simulink model "Pendulum"  (R2013a)
settings: Solver=ode1  SolverMode=SingleTasking  StartTime=0.0  StopTime=inf  FixedStep=0.01  RelTol=1e-3
InitFcn:
  | fuzzycontroller1=readfis('fuzzy1.fis');
  | fuzzycontroller2=readfis('fuzzy2.fis');
  | fuzzypid=readfis('fuzzy3.fis');
libraries: neural x91, fuzblock x9
(part 1 of 2)
settings Model: Creator=Administrator  LastModifiedBy=Administrator

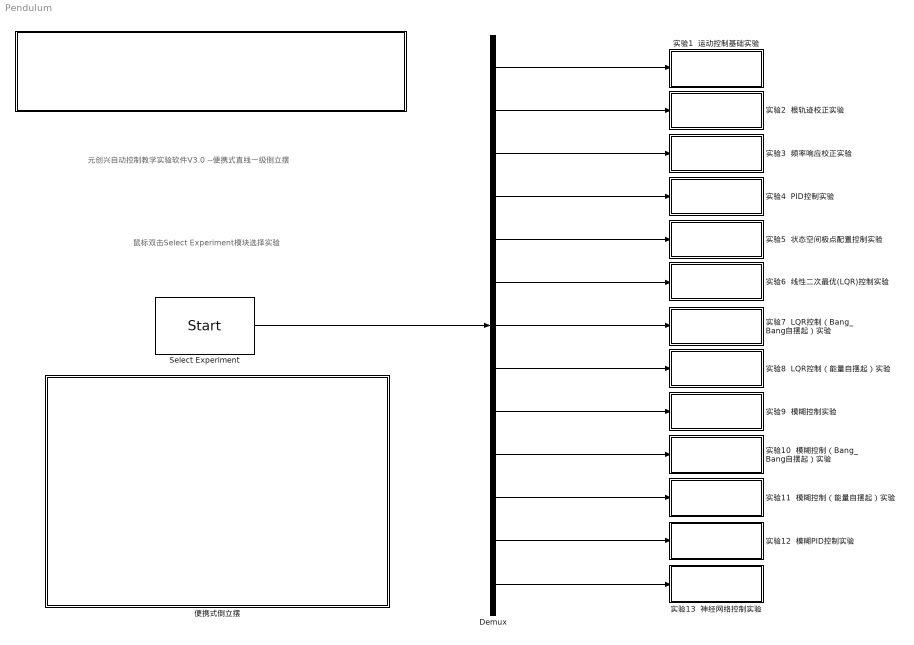
== system Pendulum ==
  note: 鼠标双击Select Experiment模块选择实验
  note: 元创兴自动控制教学实验软件V3.0
      | --便携式直线一级倒立摆
  " " : Subsystem  mask(便携式倒立摆系统实时控制程序){}
      mask help:
      | 程序版本：REI-PD-M-V3.0
      | 开发环境：Matlab2013a Simulink
      | 操作系统：Windows 7 旗舰版 32位
      | 深圳市元创兴科技有限公司
      | Copyright (C) 2015
      | 技术支持：0755-86000801
      mask Display: image('logo.PNG')
  Demux : Demux  Outputs=13
  Select Experiment : S-Function  FunctionName=Start  Parameters=ExpNum  EnableBusSupport=off  mask(SelectExperiment){ExpNum=7}
      mask prompts: ExpNum "选择实验编号："
      mask help:
      | 元创兴便携式倒立摆simulink模块：
      |
      | 便携式倒立摆可以开展以下实验：
      | 1.运动控制基础实验（编码器原理及电机运动测试）；
      | 2.根轨迹校正实验；
      | 3.频率响应校正实验；
      | 4.PID控制实验；
      | 5.状态空间极点配置控制实验；
      | 6.线性二次型最优控制实验（LQR）；
      | 7.LQR控制（Bang_Bang自摆起）实验；
      | 8.LQR控制（能量自摆起）实验；
      | 9.模糊控制实验；
      | 10.模糊控制（Bang_Bang自摆起）实验；
      | 11.模糊控制（能量自摆起）实验；
      | 12.模糊PID控制实验；
      | 13.神经网络控制实验；
      |
      | 选择实验编号后再点选启动开始实验，如果需要开展其他实验，请先停止实验后再选择。
      mask TypeOptions ExpNum: 1 | 2 | 3 | 4 | 5 | 6 | 7 | 8 | 9 | 10 | 11 | 12 | 13
      mask Display: fprintf('实验%d',ExpNum)
  便携式倒立摆 : Subsystem
      mask Display: image('Reinovo.jpg')
  实验1  运动控制基础实验 : Subsystem
  实验10  模糊控制（Bang_Bang自摆起）实验 : Subsystem  TreatAsAtomicUnit=on
  实验11  模糊控制（能量自摆起）实验 : Subsystem  TreatAsAtomicUnit=on
  实验12  模糊PID控制实验 : Subsystem  TreatAsAtomicUnit=on
  实验13  神经网络控制实验 : Subsystem  TreatAsAtomicUnit=on
  实验2  根轨迹校正实验 : Subsystem
  实验3  频率响应校正实验 : Subsystem
  实验4  PID控制实验 : Subsystem
  实验5  状态空间极点配置控制实验 : Subsystem
  实验6  线性二次最优(LQR)控制实验 : Subsystem
  实验7  LQR控制（Bang_Bang自摆起）实验 : Subsystem
  实验8  LQR控制（能量自摆起）实验 : Subsystem
  实验9  模糊控制实验 : Subsystem  TreatAsAtomicUnit=on
  wires:
  Demux/1 -> 实验1  运动控制基础实验/Enable
  Demux/2 -> 实验2  根轨迹校正实验/Enable
  Demux/3 -> 实验3  频率响应校正实验/Enable
  Demux/4 -> 实验4  PID控制实验/Enable
  Demux/5 -> 实验5  状态空间极点配置控制实验/Enable
  Demux/6 -> 实验6  线性二次最优(LQR)控制实验/Enable
  Demux/7 -> 实验7  LQR控制（Bang_Bang自摆起）实验/Enable
  Demux/8 -> 实验8  LQR控制（能量自摆起）实验/Enable
  Select Experiment/1 -> Demux/1
  Demux/9 -> 实验9  模糊控制实验/Enable
  Demux/10 -> 实验10  模糊控制（Bang_Bang自摆起）实验/Enable
  Demux/11 -> 实验11  模糊控制（能量自摆起）实验/Enable
  Demux/12 -> 实验12  模糊PID控制实验/Enable
  Demux/13 -> 实验13  神经网络控制实验/Enable

== system Pendulum/  ==

== system Pendulum/便携式倒立摆 ==

== system Pendulum/实验1  运动控制基础实验 ==
  note: 数值输入范围[-0.2~0.2] 单位m
  note: 即电机转动一圈反馈回来的脉冲数为4000
  note: 实际脉冲数
  note: 目标脉冲数
  note: 实际位移量
  note: 目标位移量
  note: 小车位置脉冲
  note: 摆杆位置脉冲
  note: 实验1 运动控制基础实验
  note: 运行前请留意小车目标位移量设置
  note: 注意：实验开始前先将小车移至导轨中间位置
  note: 1.光电编码器认知实验部分
  note: 1.摆杆编码器为500线，四倍频：500*4=2000，即摆杆旋转一圈反馈回来的脉冲数为2000
  note: 2.直流伺服电机位置控制实验
  note: 2. 电机编码器为1000线，四倍频：1000*4=4000，
  note: 转换关系：电机直径=0.0355m,周长= 0.0355*3.141592=0.1117465m,
      |   即电机转动一周小车移动的位移量=0.1117465m
  note: 电机脉冲当量=0.1117465m/4000pulse
  Enable : EnablePort
  " " : Display
  Demux : Demux  Outputs=2
  Mux : Mux  Inputs=2
  Mux1 : Mux
  小车目标位移量 : Constant  Value=0.13
  小车移动至目标位置 : S-Function  FunctionName=MoveCartPos  EnableBusSupport=off
  数字显示 : Display
  显示摆杆脉冲和角度 : Scope  NumInputPorts=2
      settings: RequirementInfo="{}  %GIDa_b12c0a95_567d_4469_aa8f_37c49eb9258f"  YMin=-5~-5  YMax=5~5
  读取两路脉冲信号 : S-Function  FunctionName=Readtwochannelpulse  Parameters=1  EnableBusSupport=off
  转换为位移 : Gain  Gain=0.1117465/4000
  转换为弧度 : Gain  Gain=2*3.1415926/2000
  转换为脉冲数 : Gain  Gain=4000/0.1117465
  wires:
  Demux/2 -> Mux/1, 显示摆杆脉冲和角度/1, 转换为弧度/1
  Demux/1 -> Mux1/4, 转换为位移/1
  读取两路脉冲信号/1 -> Demux/1
  转换为弧度/1 -> Mux/2, 显示摆杆脉冲和角度/2
  Mux/1 -> 数字显示/1
  Mux1/1 -> " "/1
  转换为位移/1 -> Mux1/2
  转换为脉冲数/1 -> Mux1/3
  小车目标位移量/1 -> 转换为脉冲数/1, Mux1/1, 小车移动至目标位置/1

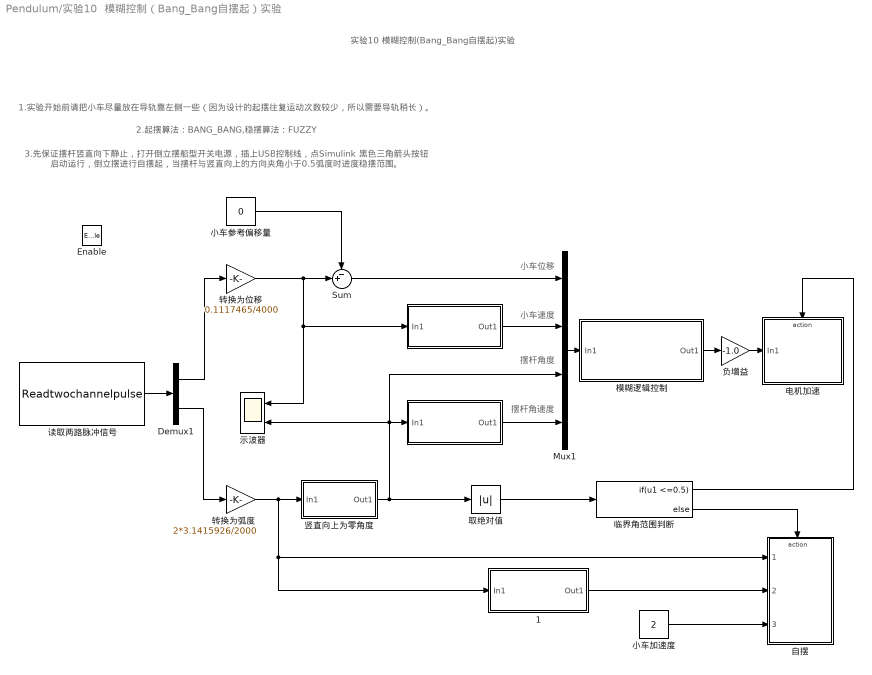
== system Pendulum/实验10  模糊控制（Bang_Bang自摆起）实验 ==
  note: 摆杆角速度
  note: 摆杆角度
  note: 小车速度
  note: 小车位移
  note: 实验10 模糊控制(Bang_Bang自摆起)实验
  note: 1.实验开始前请把小车尽量放在导轨靠左侧一些（因为设计的起摆往复运动次数较少，所以需要导轨稍长）。
  note: 3.先保证摆杆竖直向下静止，打开倒立摆船型开关电源，插上USB控制线，点Simulink 黑色三角箭头按钮
      | 启动运行，倒立摆进行自摆起，当摆杆与竖直向上的方向夹角小于0.5弧度时进度稳摆范围。
  note: 2.起摆算法：BANG_BANG,稳摆算法：FUZZY
  Enable : EnablePort
  " " : Subsystem
      mask help: 对摆杆角度求导得到摆杆角速度
      mask Display: disp('计算摆杆角速度')
  "  " : Subsystem
      mask help: 对小车位移求导得到小车速度
      mask Display: disp('计算小车速度')
  " 1" : Subsystem
      mask help: 对摆杆角度求导得到摆杆角速度
      mask Display: disp('计算摆杆角速度')
  Demux1 : Demux  Outputs=2
  Mux1 : Mux
  Sum : Sum  Inputs=-+|
  临界角范围判断 : If  IfExpression=u1 <=0.5
  取绝对值 : Abs
  小车加速度 : Constant  Value=2
  小车参考偏移量 : Constant  Value=0
  模糊逻辑控制 : Subsystem
      mask Display: disp('Fuzzy Logic Controller')
  电机加速 : Subsystem  TreatAsAtomicUnit=on
  示波器 : Scope  NumInputPorts=2
      settings: YMin=-5~-5  YMax=5~5  SaveName=ScopeData9
  竖直向上为零角度 : Subsystem
      mask help: 定义摆杆竖直向上时为零角度
      mask Display: disp('角度转换')
  自摆 : Subsystem  TreatAsAtomicUnit=on
  读取两路脉冲信号 : S-Function  FunctionName=Readtwochannelpulse  Parameters=1  EnableBusSupport=off
  负增益 : Gain  Gain=-1.0
  转换为位移 : Gain  Gain=0.1117465/4000
  转换为弧度 : Gain  Gain=2*3.1415926/2000
  wires:
  转换为位移/1 -> 示波器/1, "  "/1(In1), Sum/2
  读取两路脉冲信号/1 -> Demux1/1
  Demux1/2 -> 转换为弧度/1
  Demux1/1 -> 转换为位移/1
  小车加速度/1 -> 自摆/3("   ")
  负增益/1 -> 电机加速/1(In1)
  取绝对值/1 -> 临界角范围判断/1
  小车参考偏移量/1 -> Sum/1
  临界角范围判断/2 -> 自摆/Action
  Sum/1 -> Mux1/1
  临界角范围判断/1 -> 电机加速/Action
  模糊逻辑控制/1(Out1) -> 负增益/1
  "  "/1(Out1) -> Mux1/2
  竖直向上为零角度/1(Out1) -> 取绝对值/1, 示波器/2, " "/1(In1), Mux1/3
  " "/1(Out1) -> Mux1/4
  Mux1/1 -> 模糊逻辑控制/1(In1)
  " 1"/1(Out1) -> 自摆/2("  ")
  转换为弧度/1 -> 竖直向上为零角度/1(In1), 自摆/1(" "), " 1"/1(In1)

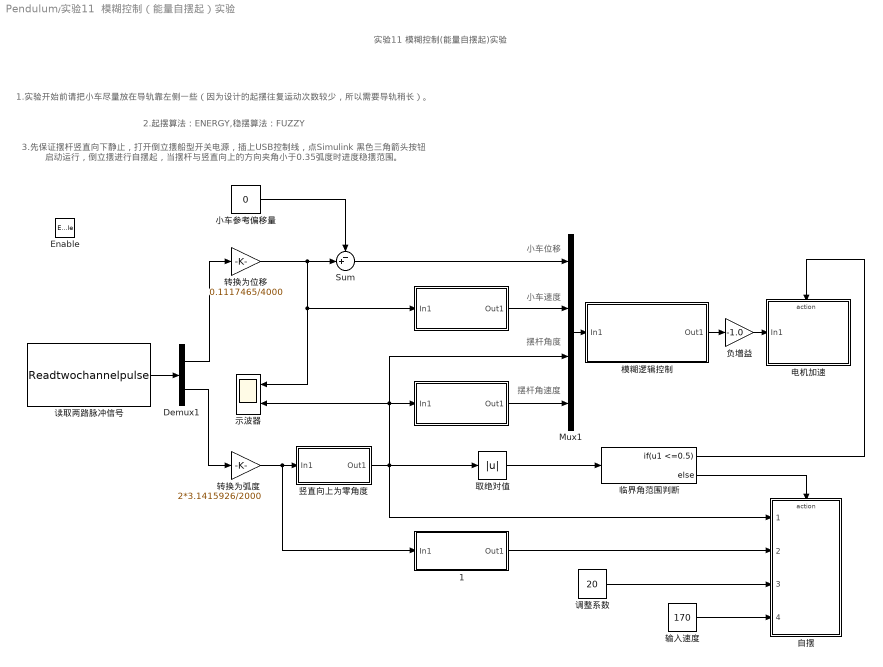
== system Pendulum/实验11  模糊控制（能量自摆起）实验 ==
  note: 摆杆角速度
  note: 摆杆角度
  note: 小车速度
  note: 小车位移
  note: 实验11 模糊控制(能量自摆起)实验
  note: 1.实验开始前请把小车尽量放在导轨靠左侧一些（因为设计的起摆往复运动次数较少，所以需要导轨稍长）。
  note: 2.起摆算法：ENERGY,稳摆算法：FUZZY
  note: 3.先保证摆杆竖直向下静止，打开倒立摆船型开关电源，插上USB控制线，点Simulink 黑色三角箭头按钮
      | 启动运行，倒立摆进行自摆起，当摆杆与竖直向上的方向夹角小于0.35弧度时进度稳摆范围。
  Enable : EnablePort
  " " : Subsystem
      mask help: 对摆杆角度求导得到摆杆角速度
      mask Display: disp('计算摆杆角速度')
  "  " : Subsystem
      mask help: 对小车位移求导得到小车速度
      mask Display: disp('计算小车速度')
  " 1" : Subsystem
      mask help: 对摆杆角度求导得到摆杆角速度
      mask Display: disp('计算摆杆角速度')
  Demux1 : Demux  Outputs=2
  Mux1 : Mux
  Sum : Sum  Inputs=-+|
  临界角范围判断 : If  IfExpression=u1 <=0.5
  取绝对值 : Abs
  小车参考偏移量 : Constant  Value=0
  模糊逻辑控制 : Subsystem
      mask Display: disp('Fuzzy Logic Controller')
  电机加速 : Subsystem  TreatAsAtomicUnit=on
  示波器 : Scope  NumInputPorts=2
      settings: YMin=-5~-5  YMax=5~5  SaveName=ScopeData10
  竖直向上为零角度 : Subsystem
      mask help: 定义摆杆竖直向上时为零角度
      mask Display: disp('角度转换')
  自摆 : Subsystem  TreatAsAtomicUnit=on
  读取两路脉冲信号 : S-Function  FunctionName=Readtwochannelpulse  Parameters=1  EnableBusSupport=off
  调整系数 : Constant  Value=20
  负增益 : Gain  Gain=-1.0
  转换为位移 : Gain  Gain=0.1117465/4000
  转换为弧度 : Gain  Gain=2*3.1415926/2000
  输入速度 : Constant  Value=170
  wires:
  转换为位移/1 -> 示波器/1, "  "/1(In1), Sum/2
  读取两路脉冲信号/1 -> Demux1/1
  Demux1/2 -> 转换为弧度/1
  Demux1/1 -> 转换为位移/1
  调整系数/1 -> 自摆/3("   ")
  负增益/1 -> 电机加速/1(In1)
  取绝对值/1 -> 临界角范围判断/1
  小车参考偏移量/1 -> Sum/1
  Sum/1 -> Mux1/1
  临界角范围判断/1 -> 电机加速/Action
  模糊逻辑控制/1(Out1) -> 负增益/1
  "  "/1(Out1) -> Mux1/2
  竖直向上为零角度/1(Out1) -> 取绝对值/1, 自摆/1(" "), 示波器/2, " "/1(In1), Mux1/3
  " "/1(Out1) -> Mux1/4
  Mux1/1 -> 模糊逻辑控制/1(In1)
  " 1"/1(Out1) -> 自摆/2("  ")
  转换为弧度/1 -> 竖直向上为零角度/1(In1), " 1"/1(In1)
  临界角范围判断/2 -> 自摆/Action
  输入速度/1 -> 自摆/4("      ")

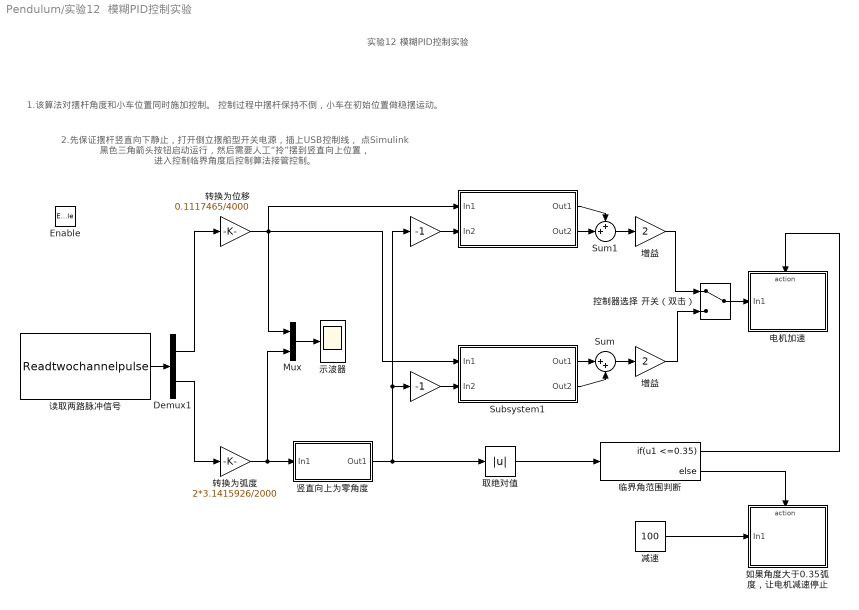
== system Pendulum/实验12  模糊PID控制实验 ==
  note: 实验12 模糊PID控制实验
  note: 1.该算法对摆杆角度和小车位置同时施加控制。
      | 控制过程中摆杆保持不倒，小车在初始位置做稳摆运动。
  note: 2.先保证摆杆竖直向下静止，打开倒立摆船型开关电源，插上USB控制线，
      | 点Simulink 黑色三角箭头按钮启动运行，然后需要人工“拎”摆到竖直向上位置，
      | 进入控制临界角度后控制算法接管控制。
  Enable : EnablePort
  " " : Gain  Gain=-1
  "  " : Gain  Gain=-1
  "     " : Subsystem
      mask Display: disp('双闭环模糊PID控制1')
  Demux1 : Demux  Outputs=2
  Mux : Mux  Inputs=2
  Subsystem1 : Subsystem
      mask Display: disp('双闭环模糊PID控制2')
  Sum : Sum  Inputs=|++
  Sum1 : Sum  Inputs=++|
  临界角范围判断 : If  IfExpression=u1 <=0.35
  减速 : Constant  Value=100
  取绝对值 : Abs
  增益 : Gain  Gain=2
  "增益 " : Gain  Gain=2
  如果角度大于0.35弧 度，让电机减速停止 : Subsystem  TreatAsAtomicUnit=on
  控制器选择 开关（双击） : ManualSwitch
  电机加速 : Subsystem  TreatAsAtomicUnit=on
  示波器 : Scope
      settings: SaveName=ScopeData11
  竖直向上为零角度 : Subsystem
      mask help: 定义摆杆竖直向上时为零角度
      mask Display: disp('角度转换')
  读取两路脉冲信号 : S-Function  FunctionName=Readtwochannelpulse  Parameters=1  EnableBusSupport=off
  转换为位移 : Gain  Gain=0.1117465/4000
  转换为弧度 : Gain  Gain=2*3.1415926/2000
  wires:
  Demux1/2 -> 转换为弧度/1
  Demux1/1 -> 转换为位移/1
  Mux/1 -> 示波器/1
  临界角范围判断/1 -> 电机加速/Action
  减速/1 -> 如果角度大于0.35弧 度，让电机减速停止/1(In1)
  转换为位移/1 -> Mux/1, Subsystem1/1(In1), "     "/1(In1)
  竖直向上为零角度/1(Out1) -> 取绝对值/1, " "/1, "  "/1
  取绝对值/1 -> 临界角范围判断/1
  读取两路脉冲信号/1 -> Demux1/1
  临界角范围判断/2 -> 如果角度大于0.35弧 度，让电机减速停止/Action
  转换为弧度/1 -> 竖直向上为零角度/1(In1), Mux/2
  控制器选择 开关（双击）/1 -> 电机加速/1(In1)
  "增益 "/1 -> 控制器选择 开关（双击）/1
  增益/1 -> 控制器选择 开关（双击）/2
  Sum/1 -> 增益/1
  " "/1 -> "     "/2(In2)
  Sum1/1 -> "增益 "/1
  "     "/2(Out2) -> Sum1/2
  "     "/1(Out1) -> Sum1/1
  "  "/1 -> Subsystem1/2(In2)
  Subsystem1/1(Out1) -> Sum/1
  Subsystem1/2(Out2) -> Sum/2

== system Pendulum/实验13  神经网络控制实验 ==
  note: 摆杆角速度
  note: 摆杆角度
  note: 小车速度
  note: 小车位移
  note: 实验13 神经网络控制实验
  note: 1.该算法对摆杆角度和小车位置同时施加控制。
      | 控制过程中摆杆保持不倒，小车在初始位置做稳摆运动。
  note: 2.先保证摆杆竖直向下静止，打开倒立摆船型开关电源，插上USB控制线，
      | 点Simulink 黑色三角箭头按钮启动运行，然后需要人工“拎”摆到竖直向上位置，
      | 进入控制临界角度后控制算法接管控制。
  Enable : EnablePort
  " " : Subsystem
      mask help: 对摆杆角度求导得到摆杆角速度
      mask Display: disp('计算摆杆角速度')
  "  " : Subsystem
      mask help: 对小车位移求导得到小车速度
      mask Display: disp('计算小车速度')
  Demux1 : Demux  Outputs=2
  Mux : Mux  Inputs=2
  Mux1 : Mux
  Sum : Sum  Inputs=-+|
  临界角范围判断 : If  IfExpression=u1 <=0.25
  减速 : Constant  Value=100
  取绝对值 : Abs
  增益 : Gain  Gain=0.8
  如果角度大于0.25弧 度，让电机减速停止 : Subsystem  TreatAsAtomicUnit=on
  小车参考偏移量 : Constant  Value=0
  电机加速 : Subsystem  TreatAsAtomicUnit=on
  示波器 : Scope
      settings: TimeRange=25000  YMin=0  YMax=3500000  SaveName=ScopeData12
  神经网络控制器 : Subsystem
      mask Display: disp('神经网络控制器')
  竖直向上为零角度 : Subsystem
      mask help: 定义摆杆竖直向上时为零角度
      mask Display: disp('角度转换')
  读取两路脉冲信号 : S-Function  FunctionName=Readtwochannelpulse  Parameters=1  EnableBusSupport=off
  转换为位移 : Gain  Gain=0.1117465/4000
  转换为弧度 : Gain  Gain=2*3.1415926/2000
  wires:
  读取两路脉冲信号/1 -> Demux1/1
  取绝对值/1 -> 临界角范围判断/1
  Mux/1 -> 示波器/1
  Demux1/1 -> 转换为位移/1
  转换为弧度/1 -> 竖直向上为零角度/1(In1), Mux/2
  Demux1/2 -> 转换为弧度/1
  竖直向上为零角度/1(Out1) -> 取绝对值/1, " "/1(In1), Mux1/3
  转换为位移/1 -> "  "/1(In1), Sum/2, Mux/1
  小车参考偏移量/1 -> Sum/1
  减速/1 -> 如果角度大于0.25弧 度，让电机减速停止/1(In1)
  临界角范围判断/2 -> 如果角度大于0.25弧 度，让电机减速停止/Action
  Sum/1 -> Mux1/1
  " "/1(Out1) -> Mux1/4
  "  "/1(Out1) -> Mux1/2
  增益/1 -> 电机加速/1(In1)
  临界角范围判断/1 -> 电机加速/Action
  神经网络控制器/1(Out1) -> 增益/1
  Mux1/1 -> 神经网络控制器/1(In1)

== system Pendulum/实验2  根轨迹校正实验 ==
  note: 实验2 根轨迹校正实验
  note: 1.该算法只对摆杆角度施加控制。
      | 控制过程中摆杆保持不倒，但小车将会左右运动直到碰到限位停止。
  note: 2.先保证摆杆竖直向下静止，打开倒立摆船型开关电源，插上USB控制线，
      | 点Simulink 黑色三角箭头按钮启动运行，然后需要人工“拎”摆到竖直向上位置，
      | 进入控制临界角度后控制算法接管控制。
  Enable : EnablePort
  Demux1 : Demux  Outputs=2
  Mux : Mux  Inputs=2
  临界角范围判断 : If  IfExpression=u1 <=0.25
  减速 : Constant  Value=100
  取绝对值 : Abs
  如果角度大于0.25弧 度，让电机减速停止 : Subsystem  TreatAsAtomicUnit=on
  根轨迹校正器 : ZeroPole  Zeros=[-7]  Poles=[-24]  Gain=[52.71]
  电机加速 : Subsystem  TreatAsAtomicUnit=on
  示波器 : Scope
  竖直向上为零角度 : Subsystem
      mask help: 定义摆杆竖直向上时为零角度
      mask Display: disp('角度转换')
  读取两路脉冲信号 : S-Function  FunctionName=Readtwochannelpulse  Parameters=1  EnableBusSupport=off
  负增益 : Gain  Gain=-1
  转换为位移 : Gain  Gain=0.1117465/4000
  转换为弧度 : Gain  Gain=2*3.1415926/2000
  wires:
  Demux1/2 -> 转换为弧度/1
  Demux1/1 -> 转换为位移/1
  读取两路脉冲信号/1 -> Demux1/1
  Mux/1 -> 示波器/1
  转换为位移/1 -> Mux/1
  转换为弧度/1 -> 竖直向上为零角度/1(In1), Mux/2
  竖直向上为零角度/1(Out1) -> 根轨迹校正器/1, 取绝对值/1
  根轨迹校正器/1 -> 负增益/1
  取绝对值/1 -> 临界角范围判断/1
  负增益/1 -> 电机加速/1(In1)
  减速/1 -> 如果角度大于0.25弧 度，让电机减速停止/1(In1)
  临界角范围判断/2 -> 如果角度大于0.25弧 度，让电机减速停止/Action
  临界角范围判断/1 -> 电机加速/Action

== system Pendulum/实验3  频率响应校正实验 ==
  note: 实验3 频率响应校正实验
  note: 1.该算法只对摆杆角度施加控制。
      | 控制过程中摆杆保持不倒，但小车将会左右运动直到碰到限位停止。
  note: 2.先保证摆杆竖直向下静止，打开倒立摆船型开关电源，插上USB控制线，
      | 点Simulink 黑色三角箭头按钮启动运行，然后需要人工“拎”摆到竖直向上位置，
      | 进入控制临界角度后控制算法接管控制。
  Enable : EnablePort
  Demux1 : Demux  Outputs=2
  Mux : Mux  Inputs=2
  临界角范围判断 : If  IfExpression=u1 <=0.25
  减速 : Constant  Value=100
  取绝对值 : Abs
  如果角度大于0.25弧 度，让电机减速停止 : Subsystem  TreatAsAtomicUnit=on
  电机加速 : Subsystem  TreatAsAtomicUnit=on
  示波器 : Scope
      settings: SaveName=ScopeData2
  竖直向上为零角度 : Subsystem
      mask help: 定义摆杆竖直向上时为零角度
      mask Display: disp('角度转换')
  读取两路脉冲信号 : S-Function  FunctionName=Readtwochannelpulse  Parameters=1  EnableBusSupport=off
  负增益 : Gain  Gain=-1
  转换为位移 : Gain  Gain=0.1117465/4000
  转换为弧度 : Gain  Gain=2*3.1415926/2000
  频率响应校正器 : ZeroPole  Zeros=[-13.535]  Poles=[-136.166]  Gain=[600]
  wires:
  Demux1/2 -> 转换为弧度/1
  Demux1/1 -> 转换为位移/1
  读取两路脉冲信号/1 -> Demux1/1
  Mux/1 -> 示波器/1
  转换为位移/1 -> Mux/1
  转换为弧度/1 -> 竖直向上为零角度/1(In1), Mux/2
  竖直向上为零角度/1(Out1) -> 取绝对值/1, 频率响应校正器/1
  频率响应校正器/1 -> 负增益/1
  取绝对值/1 -> 临界角范围判断/1
  负增益/1 -> 电机加速/1(In1)
  减速/1 -> 如果角度大于0.25弧 度，让电机减速停止/1(In1)
  临界角范围判断/2 -> 如果角度大于0.25弧 度，让电机减速停止/Action
  临界角范围判断/1 -> 电机加速/Action

== system Pendulum/实验4  PID控制实验 ==
  note: 实验4 PID控制实验
  note: 2.双闭环PID控制器对摆杆角度和小车位置同时施加控制。
      | 控制过程中摆杆保持不倒，小车在初始位置做稳摆运动。
  note: 3.先保证摆杆竖直向下静止，打开倒立摆船型开关电源，插上USB控制线，
      | 点Simulink 黑色三角箭头按钮启动运行，然后需要人工“拎”摆到竖直向上位置，
      | 进入控制临界角度后控制算法接管控制。
  note: 1.单闭环PID控制器只对摆杆角度施加控制。
      | 控制过程中摆杆保持不倒，但小车将会左右运动直到碰到限位停止。
  Enable : EnablePort
  Demux1 : Demux  Outputs=2
  Gain : Gain  Gain=-1
  Mux : Mux  Inputs=2
  Sum : Sum  Inputs=|++
  临界角范围判断 : If  IfExpression=u1 <=0.25
  减速 : Constant  Value=100
  取绝对值 : Abs
  只对摆杆角度施加控制 : Subsystem
      mask Display: disp('单闭环PID控制器')
  增益 : Gain  Gain=14.5
  如果角度大于0.25弧 度，让电机减速停止 : Subsystem  TreatAsAtomicUnit=on
  对摆杆角度和小车 位置同时施加控制 : Subsystem
      mask Display: disp('双闭环PID控制器')
  控制器选择 开关（双击） : ManualSwitch  CurrentSetting=0
  电机加速 : Subsystem  TreatAsAtomicUnit=on
  示波器 : Scope
      settings: SaveName=ScopeData3
  竖直向上为零角度 : Subsystem
      mask help: 定义摆杆竖直向上时为零角度
      mask Display: disp('角度转换')
  读取两路脉冲信号 : S-Function  FunctionName=Readtwochannelpulse  Parameters=1  EnableBusSupport=off
  负增益 : Gain  Gain=-1
  转换为位移 : Gain  Gain=0.1117465/4000
  转换为弧度 : Gain  Gain=2*3.1415926/2000
  wires:
  Demux1/2 -> 转换为弧度/1
  Demux1/1 -> 转换为位移/1
  Mux/1 -> 示波器/1
  临界角范围判断/1 -> 电机加速/Action
  减速/1 -> 如果角度大于0.25弧 度，让电机减速停止/1(In1)
  转换为位移/1 -> 对摆杆角度和小车 位置同时施加控制/1(In3), Mux/1
  竖直向上为零角度/1(Out1) -> 取绝对值/1, Gain/1, 只对摆杆角度施加控制/1(In1)
  取绝对值/1 -> 临界角范围判断/1
  读取两路脉冲信号/1 -> Demux1/1
  临界角范围判断/2 -> 如果角度大于0.25弧 度，让电机减速停止/Action
  转换为弧度/1 -> 竖直向上为零角度/1(In1), Mux/2
  只对摆杆角度施加控制/1(Out1) -> 负增益/1
  控制器选择 开关（双击）/1 -> 电机加速/1(In1)
  负增益/1 -> 控制器选择 开关（双击）/1
  增益/1 -> 控制器选择 开关（双击）/2
  Sum/1 -> 增益/1
  对摆杆角度和小车 位置同时施加控制/1(Out3) -> Sum/1
  对摆杆角度和小车 位置同时施加控制/2(Out2) -> Sum/2
  Gain/1 -> 对摆杆角度和小车 位置同时施加控制/2(In2)

== system Pendulum/实验5  状态空间极点配置控制实验 ==
  note: 摆杆角速度
  note: 摆杆角度
  note: 小车速度
  note: 小车位移
  note: 实验5 状态空间极点配置控制实验
  note: 1.该算法对摆杆角度和小车位置同时施加控制。
      | 控制过程中摆杆保持不倒，小车在初始位置做稳摆运动。
  note: 2.先保证摆杆竖直向下静止，打开倒立摆船型开关电源，插上USB控制线，
      | 点Simulink 黑色三角箭头按钮启动运行，然后需要人工“拎”摆到竖直向上位置，
      | 进入控制临界角度后控制算法接管控制。
  Enable : EnablePort
  " " : Subsystem
      mask help: 对摆杆角度求导得到摆杆角速度
      mask Display: disp('计算摆杆角速度')
  "  " : Subsystem
      mask help: 对小车位移求导得到小车速度
      mask Display: disp('计算小车速度')
  "   " : Subsystem  mask{K1=-26.667, K2=-12, K3=46.1723, K4=5.8804}
      mask help: LQR控制器
      mask Display: disp('状态空间极点配置控制器')
  Demux1 : Demux  Outputs=2
  Mux : Mux  Inputs=2
  Mux1 : Mux
  Sum : Sum  Inputs=-+|
  临界角范围判断 : If  IfExpression=u1 <=0.25
  减速 : Constant  Value=100
  取绝对值 : Abs
  如果角度大于0.25弧 度，让电机减速停止 : Subsystem  TreatAsAtomicUnit=on
  小车参考偏移量 : Constant  Value=0
  电机加速 : Subsystem  TreatAsAtomicUnit=on
  示波器 : Scope
      settings: SaveName=ScopeData4
  竖直向上为零角度 : Subsystem
      mask help: 定义摆杆竖直向上时为零角度
      mask Display: disp('角度转换')
  读取两路脉冲信号 : S-Function  FunctionName=Readtwochannelpulse  Parameters=1  EnableBusSupport=off
  负增益 : Gain  Gain=-1.0
  转换为位移 : Gain  Gain=0.1117465/4000
  转换为弧度 : Gain  Gain=2*3.1415926/2000
  wires:
  读取两路脉冲信号/1 -> Demux1/1
  取绝对值/1 -> 临界角范围判断/1
  Mux/1 -> 示波器/1
  Demux1/1 -> 转换为位移/1
  转换为弧度/1 -> 竖直向上为零角度/1(In1), Mux/2
  Demux1/2 -> 转换为弧度/1
  竖直向上为零角度/1(Out1) -> 取绝对值/1, " "/1(In1), Mux1/3
  转换为位移/1 -> "  "/1(In1), Sum/2, Mux/1
  小车参考偏移量/1 -> Sum/1
  减速/1 -> 如果角度大于0.25弧 度，让电机减速停止/1(In1)
  临界角范围判断/2 -> 如果角度大于0.25弧 度，让电机减速停止/Action
  Sum/1 -> Mux1/1
  " "/1(Out1) -> Mux1/4
  "  "/1(Out1) -> Mux1/2
  Mux1/1 -> "   "/1(In1)
  "   "/1(Out1) -> 负增益/1
  负增益/1 -> 电机加速/1(In1)
  临界角范围判断/1 -> 电机加速/Action

== system Pendulum/实验6  线性二次最优(LQR)控制实验 ==
  note: 摆杆角速度
  note: 摆杆角度
  note: 小车速度
  note: 小车位移
  note: 实验6 线性二次最优控制实验
  note: 1.该算法对摆杆角度和小车位置同时施加控制。
      | 控制过程中摆杆保持不倒，小车在初始位置做稳摆运动。
  note: 2.先保证摆杆竖直向下静止，打开倒立摆船型开关电源，插上USB控制线，
      | 点Simulink 黑色三角箭头按钮启动运行，然后需要人工“拎”摆到竖直向上位置，
      | 进入控制临界角度后控制算法接管控制。
  Enable : EnablePort
  " " : Subsystem
      mask help: 对摆杆角度求导得到摆杆角速度
      mask Display: disp('计算摆杆角速度')
  "  " : Subsystem
      mask help: 对小车位移求导得到小车速度
      mask Display: disp('计算小车速度')
  Demux1 : Demux  Outputs=2
  Mux : Mux  Inputs=2
  Mux1 : Mux
  Sum : Sum  Inputs=-+|
  临界角范围判断 : If  IfExpression=u1 <=0.25
  减速 : Constant  Value=100
  取绝对值 : Abs
  如果角度大于0.25弧 度，让电机减速停止 : Subsystem  TreatAsAtomicUnit=on
  小车参考偏移量 : Constant  Value=0
  电机加速 : Subsystem  TreatAsAtomicUnit=on
  示波器 : Scope
      settings: SaveName=ScopeData5
  竖直向上为零角度 : Subsystem
      mask help: 定义摆杆竖直向上时为零角度
      mask Display: disp('角度转换')
  线性二次最优控制器 : Subsystem  mask{K1=-10, K2=-7.4869, K3=37.2688, K4=4.6349}
      mask help: LQR控制器
      mask Display: disp('LQR控制器')
  读取两路脉冲信号 : S-Function  FunctionName=Readtwochannelpulse  Parameters=1  EnableBusSupport=off
  负增益 : Gain  Gain=-1.0
  转换为位移 : Gain  Gain=0.1117465/4000
  转换为弧度 : Gain  Gain=2*3.1415926/2000
  wires:
  转换为位移/1 -> "  "/1(In1), Sum/2, Mux/1
  Mux/1 -> 示波器/1
  读取两路脉冲信号/1 -> Demux1/1
  Demux1/2 -> 转换为弧度/1
  Demux1/1 -> 转换为位移/1
  减速/1 -> 如果角度大于0.25弧 度，让电机减速停止/1(In1)
  负增益/1 -> 电机加速/1(In1)
  取绝对值/1 -> 临界角范围判断/1
  Mux1/1 -> 线性二次最优控制器/1(In1)
  小车参考偏移量/1 -> Sum/1
  临界角范围判断/2 -> 如果角度大于0.25弧 度，让电机减速停止/Action
  转换为弧度/1 -> 竖直向上为零角度/1(In1), Mux/2
  Sum/1 -> Mux1/1
  临界角范围判断/1 -> 电机加速/Action
  线性二次最优控制器/1(Out1) -> 负增益/1
  "  "/1(Out1) -> Mux1/2
  竖直向上为零角度/1(Out1) -> 取绝对值/1, " "/1(In1), Mux1/3
  " "/1(Out1) -> Mux1/4

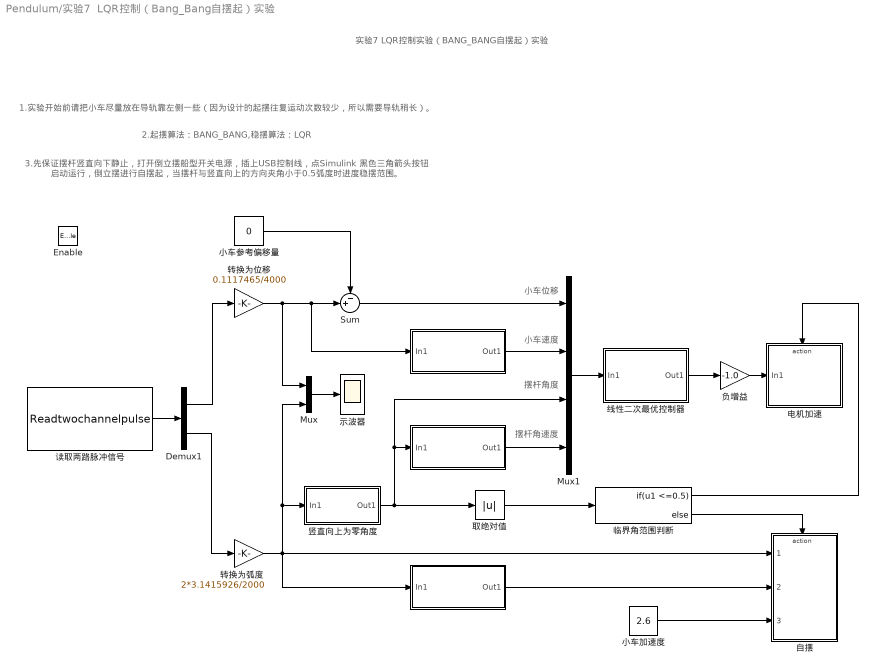
== system Pendulum/实验7  LQR控制（Bang_Bang自摆起）实验 ==
  note: 摆杆角速度
  note: 摆杆角度
  note: 小车速度
  note: 小车位移
  note: 实验7 LQR控制实验（BANG_BANG自摆起）实验
  note: 1.实验开始前请把小车尽量放在导轨靠左侧一些（因为设计的起摆往复运动次数较少，所以需要导轨稍长）。
  note: 3.先保证摆杆竖直向下静止，打开倒立摆船型开关电源，插上USB控制线，点Simulink 黑色三角箭头按钮
      | 启动运行，倒立摆进行自摆起，当摆杆与竖直向上的方向夹角小于0.5弧度时进度稳摆范围。
  note: 2.起摆算法：BANG_BANG,稳摆算法：LQR
  Enable : EnablePort
  " " : Subsystem
      mask help: 对摆杆角度求导得到摆杆角速度
      mask Display: disp('计算摆杆角速度')
  "  " : Subsystem
      mask help: 对小车位移求导得到小车速度
      mask Display: disp('计算小车速度')
  "       " : Subsystem
      mask help: 对摆杆角度求导得到摆杆角速度
      mask Display: disp('计算摆杆角速度')
  Demux1 : Demux  Outputs=2
  Mux : Mux  Inputs=2
  Mux1 : Mux
  Sum : Sum  Inputs=-+|
  临界角范围判断 : If  IfExpression=u1 <=0.5
  取绝对值 : Abs
  小车加速度 : Constant  Value=2.6
  小车参考偏移量 : Constant  Value=0
  电机加速 : Subsystem  TreatAsAtomicUnit=on
  示波器 : Scope
      settings: SaveName=ScopeData6
  竖直向上为零角度 : Subsystem
      mask help: 定义摆杆竖直向上时为零角度
      mask Display: disp('角度转换')
  线性二次最优控制器 : Subsystem  mask{K1=-10, K2=-7.4869, K3=37.2688, K4=4.6349}
      mask help: LQR控制器
      mask Display: disp('LQR控制器')
  自摆 : Subsystem  TreatAsAtomicUnit=on
  读取两路脉冲信号 : S-Function  FunctionName=Readtwochannelpulse  Parameters=1  EnableBusSupport=off
  负增益 : Gain  Gain=-1.0
  转换为位移 : Gain  Gain=0.1117465/4000
  转换为弧度 : Gain  Gain=2*3.1415926/2000
  wires:
  转换为位移/1 -> "  "/1(In1), Sum/2, Mux/1
  读取两路脉冲信号/1 -> Demux1/1
  Demux1/2 -> 转换为弧度/1
  取绝对值/1 -> 临界角范围判断/1
  " "/1(Out1) -> Mux1/4
  Mux/1 -> 示波器/1
  竖直向上为零角度/1(Out1) -> 取绝对值/1, " "/1(In1), Mux1/3
  Sum/1 -> Mux1/1
  负增益/1 -> 电机加速/1(In1)
  转换为弧度/1 -> 竖直向上为零角度/1(In1), Mux/2, 自摆/1(" "), "       "/1(In1)
  Demux1/1 -> 转换为位移/1
  Mux1/1 -> 线性二次最优控制器/1(In1)
  小车参考偏移量/1 -> Sum/1
  "  "/1(Out1) -> Mux1/2
  线性二次最优控制器/1(Out1) -> 负增益/1
  临界角范围判断/1 -> 电机加速/Action
  临界角范围判断/2 -> 自摆/Action
  "       "/1(Out1) -> 自摆/2("  ")
  小车加速度/1 -> 自摆/3("   ")

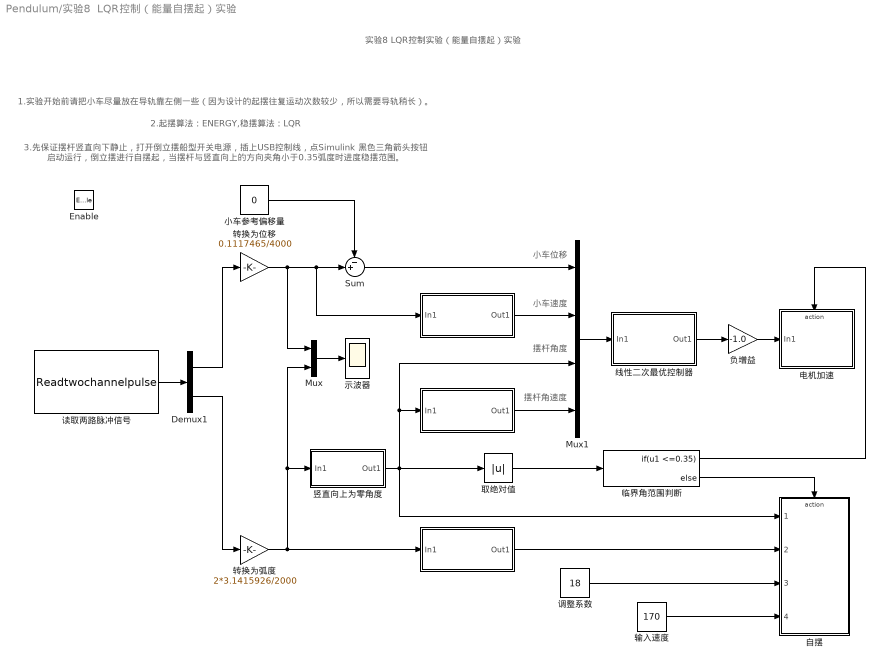
== system Pendulum/实验8  LQR控制（能量自摆起）实验 ==
  note: 摆杆角速度
  note: 摆杆角度
  note: 小车速度
  note: 小车位移
  note: 实验8 LQR控制实验（能量自摆起）实验
  note: 1.实验开始前请把小车尽量放在导轨靠左侧一些（因为设计的起摆往复运动次数较少，所以需要导轨稍长）。
  note: 2.起摆算法：ENERGY,稳摆算法：LQR
  note: 3.先保证摆杆竖直向下静止，打开倒立摆船型开关电源，插上USB控制线，点Simulink 黑色三角箭头按钮
      | 启动运行，倒立摆进行自摆起，当摆杆与竖直向上的方向夹角小于0.35弧度时进度稳摆范围。
  Enable : EnablePort
  " " : Subsystem
      mask help: 对摆杆角度求导得到摆杆角速度
      mask Display: disp('计算摆杆角速度')
  "  " : Subsystem
      mask help: 对小车位移求导得到小车速度
      mask Display: disp('计算小车速度')
  "       " : Subsystem
      mask help: 对摆杆角度求导得到摆杆角速度
      mask Display: disp('计算摆杆角速度')
  Demux1 : Demux  Outputs=2
  Mux : Mux  Inputs=2
  Mux1 : Mux
  Sum : Sum  Inputs=-+|
  临界角范围判断 : If  IfExpression=u1 <=0.35
  取绝对值 : Abs
  小车参考偏移量 : Constant  Value=0
  电机加速 : Subsystem  TreatAsAtomicUnit=on
  示波器 : Scope
      settings: TimeRange=10  SaveName=ScopeData7
  竖直向上为零角度 : Subsystem
      mask help: 定义摆杆竖直向上时为零角度
      mask Display: disp('角度转换')
  线性二次最优控制器 : Subsystem  mask{K1=-10, K2=-7.4869, K3=37.2688, K4=4.6349}
      mask help: LQR控制器
      mask Display: disp('LQR控制器')
  自摆 : Subsystem  TreatAsAtomicUnit=on
  读取两路脉冲信号 : S-Function  FunctionName=Readtwochannelpulse  Parameters=1  EnableBusSupport=off
  调整系数 : Constant  Value=18
  负增益 : Gain  Gain=-1.0
  转换为位移 : Gain  Gain=0.1117465/4000
  转换为弧度 : Gain  Gain=2*3.1415926/2000
  输入速度 : Constant  Value=170
  wires:
  线性二次最优控制器/1(Out1) -> 负增益/1
  小车参考偏移量/1 -> Sum/1
  负增益/1 -> 电机加速/1(In1)
  Mux1/1 -> 线性二次最优控制器/1(In1)
  竖直向上为零角度/1(Out1) -> 自摆/1(" "), 取绝对值/1, " "/1(In1), Mux1/3
  Demux1/1 -> 转换为位移/1
  Mux/1 -> 示波器/1
  转换为弧度/1 -> 竖直向上为零角度/1(In1), Mux/2, "       "/1(In1)
  "       "/1(Out1) -> 自摆/2("  ")
  临界角范围判断/2 -> 自摆/Action
  调整系数/1 -> 自摆/3("   ")
  " "/1(Out1) -> Mux1/4
  临界角范围判断/1 -> 电机加速/Action
  取绝对值/1 -> 临界角范围判断/1
  Sum/1 -> Mux1/1
  "  "/1(Out1) -> Mux1/2
  Demux1/2 -> 转换为弧度/1
  转换为位移/1 -> "  "/1(In1), Sum/2, Mux/1
  读取两路脉冲信号/1 -> Demux1/1
  输入速度/1 -> 自摆/4("      ")

== system Pendulum/实验9  模糊控制实验 ==
  note: 摆杆角速度
  note: 摆杆角度
  note: 小车速度
  note: 小车位移
  note: 实验9 模糊控制实验
  note: 2.先保证摆杆竖直向下静止，打开倒立摆船型开关电源，插上USB控制线，
      | 点Simulink 黑色三角箭头按钮启动运行，然后需要人工“拎”摆到竖直向上位置，
      | 进入控制临界角度后控制算法接管控制。
  note: 1.该算法对摆杆角度和小车位置同时施加控制。
      | 控制过程中摆杆保持不倒，小车在初始位置做稳摆运动。
  Enable : EnablePort
  " " : Subsystem
      mask help: 对摆杆角度求导得到摆杆角速度
      mask Display: disp('计算摆杆角速度')
  "  " : Subsystem
      mask help: 对小车位移求导得到小车速度
      mask Display: disp('计算小车速度')
  Demux1 : Demux  Outputs=2
  Mux1 : Mux
  Sum : Sum  Inputs=-+|
  临界角范围判断 : If  IfExpression=u1 <=0.25
  减速 : Constant  Value=100
  取绝对值 : Abs
  小车参考偏移量 : Constant  Value=0
  模糊逻辑控制 : Subsystem
      mask Display: disp('Fuzzy Logic Controller')
  电机停止 : Subsystem  TreatAsAtomicUnit=on
  电机加速 : Subsystem  TreatAsAtomicUnit=on
  示波器 : Scope  NumInputPorts=2
      settings: YMin=-5~-5  YMax=5~5  SaveName=ScopeData8
  竖直向上为零角度 : Subsystem
      mask help: 定义摆杆竖直向上时为零角度
      mask Display: disp('角度转换')
  读取两路脉冲信号 : S-Function  FunctionName=Readtwochannelpulse  Parameters=1  EnableBusSupport=off
  负增益 : Gain  Gain=-1.0
  转换为位移 : Gain  Gain=0.1117465/4000
  转换为弧度 : Gain  Gain=2*3.1415926/2000
  wires:
  转换为位移/1 -> 示波器/1, "  "/1(In1), Sum/2
  读取两路脉冲信号/1 -> Demux1/1
  Demux1/2 -> 转换为弧度/1
  Demux1/1 -> 转换为位移/1
  减速/1 -> 电机停止/1(In1)
  负增益/1 -> 电机加速/1(In1)
  取绝对值/1 -> 临界角范围判断/1
  小车参考偏移量/1 -> Sum/1
  临界角范围判断/2 -> 电机停止/Action
  转换为弧度/1 -> 竖直向上为零角度/1(In1)
  Sum/1 -> Mux1/1
  临界角范围判断/1 -> 电机加速/Action
  模糊逻辑控制/1(Out1) -> 负增益/1
  "  "/1(Out1) -> Mux1/2
  竖直向上为零角度/1(Out1) -> 取绝对值/1, 示波器/2, " "/1(In1), Mux1/3
  " "/1(Out1) -> Mux1/4
  Mux1/1 -> 模糊逻辑控制/1(In1)

== system Pendulum/实验10  模糊控制（Bang_Bang自摆起）实验/  ==
  In1 : Inport
  Discrete Zero-Pole : DiscreteZeroPole  Poles=[0]  Gain=1  SampleTime=0.01
  Gain : Gain  Gain=1/0.01
  Out1 : Outport
  wires:
  Gain/1 -> Out1/1
  Discrete Zero-Pole/1 -> Gain/1
  In1/1 -> Discrete Zero-Pole/1

== system Pendulum/实验10  模糊控制（Bang_Bang自摆起）实验/   ==
  In1 : Inport
  Discrete Zero-Pole : DiscreteZeroPole  Poles=[0]  Gain=1  SampleTime=0.01
  Gain : Gain  Gain=1/0.01
  Out1 : Outport
  wires:
  Gain/1 -> Out1/1
  Discrete Zero-Pole/1 -> Gain/1
  In1/1 -> Discrete Zero-Pole/1

== system Pendulum/实验10  模糊控制（Bang_Bang自摆起）实验/ 1 ==
  In1 : Inport
  Discrete Zero-Pole : DiscreteZeroPole  Poles=[0]  Gain=1  SampleTime=0.01
  Gain : Gain  Gain=1/0.01
  Out1 : Outport
  wires:
  Gain/1 -> Out1/1
  Discrete Zero-Pole/1 -> Gain/1
  In1/1 -> Discrete Zero-Pole/1

== system Pendulum/实验10  模糊控制（Bang_Bang自摆起）实验/模糊逻辑控制 ==
  note: 本实验提供两个模糊控制器，你可以通过双击上面的手动开关选择模糊控制器1或者模糊控制器2，然后比较实验效果
  In1 : Inport
  Demux : Demux
  Fuzzy Logic Controller1 : fuzblock/Fuzzy Logic  Controller  fis=fuzzycontroller1
  Fuzzy Logic Controller2 : fuzblock/Fuzzy Logic  Controller  fis=fuzzycontroller2
  Gain : Gain  Gain=[-10.000 37.2688]  Multiplication=Matrix(K*u) (u vector)
  Gain2 : Gain  Gain=[-7.4869 4.6349]  Multiplication=Matrix(K*u) (u vector)
  Mux : Mux  Inputs=2
  Mux1 : Mux  Inputs=2
  Mux2 : Mux  Inputs=2
  控制器选择 开关（双击） : ManualSwitch  CurrentSetting=0
  比例因子 清晰化 : Gain  Gain=39.5790
  比例因子 清晰化1 : Gain  Gain=39.5790
  量化因子 模糊化 : Gain  Gain=1/39.5790
  量化因子 模糊化1 : Gain  Gain=1/39.5790
  Out1 : Outport
  wires:
  Mux1/1 -> Gain2/1
  Gain/1 -> Mux2/1
  Gain2/1 -> Mux2/2
  Demux/3 -> Mux/2
  量化因子 模糊化/1 -> Fuzzy Logic Controller1/1
  Fuzzy Logic Controller1/1 -> 比例因子 清晰化/1
  In1/1 -> Demux/1
  Mux2/1 -> 量化因子 模糊化1/1, 量化因子 模糊化/1
  Demux/1 -> Mux/1
  Demux/4 -> Mux1/2
  Demux/2 -> Mux1/1
  Mux/1 -> Gain/1
  量化因子 模糊化1/1 -> Fuzzy Logic Controller2/1
  Fuzzy Logic Controller2/1 -> 比例因子 清晰化1/1
  比例因子 清晰化1/1 -> 控制器选择 开关（双击）/2
  控制器选择 开关（双击）/1 -> Out1/1
  比例因子 清晰化/1 -> 控制器选择 开关（双击）/1

== system Pendulum/实验10  模糊控制（Bang_Bang自摆起）实验/电机加速 ==
  In1 : Inport
  Action Port : ActionPort  ActionType=then
  Display : Display
  S-Function : S-Function  FunctionName=SetMotorAcc  EnableBusSupport=off
  wires:
  In1/1 -> S-Function/1
  S-Function/1 -> Display/1

== system Pendulum/实验10  模糊控制（Bang_Bang自摆起）实验/竖直向上为零角度 ==
  In1 : Inport
  Constant : Constant  Value=-3.1415926
  Constant1 : Constant  Value=3.1415926
  Sum : Sum  Inputs=|++
  Switch : Switch
  Out1 : Outport
  wires:
  Switch/1 -> Sum/1
  Constant/1 -> Switch/1
  Sum/1 -> Out1/1
  In1/1 -> Sum/2, Switch/2
  Constant1/1 -> Switch/3

== system Pendulum/实验10  模糊控制（Bang_Bang自摆起）实验/自摆 ==
  " " : Inport
  "  " : Inport  Port=2
  "   " : Inport  Port=3
  Action Port : ActionPort  ActionType=else
  S-Function : S-Function  FunctionName=BangBangSwingUp  EnableBusSupport=off
      mask Display:
      | port_label('input',1,'ANG')
      | port_label('input',2,'VEL')
      | port_label('input',3,'ACC')
  wires:
  " "/1 -> S-Function/1
  "  "/1 -> S-Function/2
  "   "/1 -> S-Function/3

== system Pendulum/实验11  模糊控制（能量自摆起）实验/  ==
  In1 : Inport
  Discrete Zero-Pole : DiscreteZeroPole  Poles=[0]  Gain=1  SampleTime=0.01
  Gain : Gain  Gain=1/0.01
  Out1 : Outport
  wires:
  Gain/1 -> Out1/1
  Discrete Zero-Pole/1 -> Gain/1
  In1/1 -> Discrete Zero-Pole/1

== system Pendulum/实验11  模糊控制（能量自摆起）实验/   ==
  In1 : Inport
  Discrete Zero-Pole : DiscreteZeroPole  Poles=[0]  Gain=1  SampleTime=0.01
  Gain : Gain  Gain=1/0.01
  Out1 : Outport
  wires:
  Gain/1 -> Out1/1
  Discrete Zero-Pole/1 -> Gain/1
  In1/1 -> Discrete Zero-Pole/1

== system Pendulum/实验11  模糊控制（能量自摆起）实验/ 1 ==
  In1 : Inport
  Discrete Zero-Pole : DiscreteZeroPole  Poles=[0]  Gain=1  SampleTime=0.01
  Gain : Gain  Gain=1/0.01
  Out1 : Outport
  wires:
  Gain/1 -> Out1/1
  Discrete Zero-Pole/1 -> Gain/1
  In1/1 -> Discrete Zero-Pole/1

== system Pendulum/实验11  模糊控制（能量自摆起）实验/模糊逻辑控制 ==
  note: 本实验提供两个模糊控制器，你可以通过双击上面的手动开关选择模糊控制器1或者模糊控制器2，然后比较实验效果
  In1 : Inport
  Demux : Demux
  Fuzzy Logic Controller1 : fuzblock/Fuzzy Logic  Controller  fis=fuzzycontroller1
  Fuzzy Logic Controller2 : fuzblock/Fuzzy Logic  Controller  fis=fuzzycontroller2
  Gain : Gain  Gain=[-10.000 37.2688]  Multiplication=Matrix(K*u) (u vector)
  Gain2 : Gain  Gain=[-7.4869 4.6349]  Multiplication=Matrix(K*u) (u vector)
  Mux : Mux  Inputs=2
  Mux1 : Mux  Inputs=2
  Mux2 : Mux  Inputs=2
  控制器选择 开关（双击） : ManualSwitch  CurrentSetting=0
  比例因子 清晰化 : Gain  Gain=39.5790
  比例因子 清晰化1 : Gain  Gain=39.5790
  量化因子 模糊化 : Gain  Gain=1/39.5790
  量化因子 模糊化1 : Gain  Gain=1/39.5790
  Out1 : Outport
  wires:
  Mux1/1 -> Gain2/1
  Gain/1 -> Mux2/1
  Gain2/1 -> Mux2/2
  Demux/3 -> Mux/2
  量化因子 模糊化/1 -> Fuzzy Logic Controller1/1
  Fuzzy Logic Controller1/1 -> 比例因子 清晰化/1
  In1/1 -> Demux/1
  Mux2/1 -> 量化因子 模糊化1/1, 量化因子 模糊化/1
  Demux/1 -> Mux/1
  Demux/4 -> Mux1/2
  Demux/2 -> Mux1/1
  Mux/1 -> Gain/1
  量化因子 模糊化1/1 -> Fuzzy Logic Controller2/1
  Fuzzy Logic Controller2/1 -> 比例因子 清晰化1/1
  比例因子 清晰化1/1 -> 控制器选择 开关（双击）/2
  控制器选择 开关（双击）/1 -> Out1/1
  比例因子 清晰化/1 -> 控制器选择 开关（双击）/1

== system Pendulum/实验11  模糊控制（能量自摆起）实验/电机加速 ==
  In1 : Inport
  Action Port : ActionPort  ActionType=then
  Display : Display
  S-Function : S-Function  FunctionName=SetMotorAcc  EnableBusSupport=off
  wires:
  In1/1 -> S-Function/1
  S-Function/1 -> Display/1

== system Pendulum/实验11  模糊控制（能量自摆起）实验/竖直向上为零角度 ==
  In1 : Inport
  Constant : Constant  Value=-3.1415926
  Constant1 : Constant  Value=3.1415926
  Sum : Sum  Inputs=|++
  Switch : Switch
  Out1 : Outport
  wires:
  Switch/1 -> Sum/1
  Constant/1 -> Switch/1
  Sum/1 -> Out1/1
  In1/1 -> Sum/2, Switch/2
  Constant1/1 -> Switch/3

== system Pendulum/实验11  模糊控制（能量自摆起）实验/自摆 ==
  " " : Inport
  "  " : Inport  Port=2
  "   " : Inport  Port=3
  "      " : Inport  Port=4
  Action Port : ActionPort  ActionType=else
  能量自摆 : S-Function  FunctionName=EnergySwingUp  EnableBusSupport=off  mask(EnergySwingUp){}
      mask help:
      | 元创兴便携式倒立摆simulink模块：
      |
      | 能量自摆起算法
      | 输入参数有四个：
      | 1.摆杆角度
      | 2.摆杆速度
      | 3.调整系数
      | 4.输入速度
      mask Display:
      | disp('EnergySwingUp')
      | port_label('input',1,'ANG')
      | port_label('input',2,'VEL')
      | port_label('input',3,'RAT')
      | port_label('input',4,'ACC')
  wires:
  " "/1 -> 能量自摆/1
  "  "/1 -> 能量自摆/2
  "   "/1 -> 能量自摆/3
  "      "/1 -> 能量自摆/4

== system Pendulum/实验12  模糊PID控制实验/      ==
  In1 : Inport
  In2 : Inport  Port=2
  D1 : Display
  D2 : Display
  P1 : Display
  P2 : Display
  PID1 : Subsystem
      mask Display: disp('小车位置模糊PID校正器')
  PID2 : Subsystem
      mask Display: disp('摆杆角度模糊PID校正器')
  Out1 : Outport
  Out2 : Outport  Port=2
  wires:
  PID2/2(Out3) -> P2/1
  In2/1 -> PID2/1(In1)
  In1/1 -> PID1/1(In2)
  PID2/1(Out1) -> Out2/1
  PID1/3(Out4) -> D1/1
  PID2/3(Out4) -> D2/1
  PID1/1(Out2) -> Out1/1
  PID1/2(Out3) -> P1/1

== system Pendulum/实验12  模糊PID控制实验/Subsystem1 ==
  In1 : Inport
  In2 : Inport  Port=2
  D1 : Display
  D2 : Display
  P1 : Display
  P2 : Display
  PID1 : Subsystem
      mask Display: disp('小车位置模糊PID校正器')
  PID2 : Subsystem
      mask Display: disp('摆杆角度模糊PID校正器')
  Out1 : Outport
  Out2 : Outport  Port=2
  wires:
  PID2/2(Out3) -> P2/1
  In2/1 -> PID2/1(In1)
  In1/1 -> PID1/1(In2)
  PID2/1(Out1) -> Out2/1
  PID1/3(Out4) -> D1/1
  PID2/3(Out4) -> D2/1
  PID1/1(Out2) -> Out1/1
  PID1/2(Out3) -> P1/1

== system Pendulum/实验12  模糊PID控制实验/如果角度大于0.35弧 度，让电机减速停止 ==
  In1 : Inport
  Action Port : ActionPort  ActionType=else
  S-Function : S-Function  FunctionName=SetStop  EnableBusSupport=off
  wires:
  In1/1 -> S-Function/1

== system Pendulum/实验12  模糊PID控制实验/电机加速 ==
  In1 : Inport
  Action Port : ActionPort  ActionType=then
  Display : Display
  S-Function : S-Function  FunctionName=SetMotorAcc  EnableBusSupport=off
  wires:
  In1/1 -> S-Function/1
  S-Function/1 -> Display/1

== system Pendulum/实验12  模糊PID控制实验/竖直向上为零角度 ==
  In1 : Inport
  Constant : Constant  Value=-3.1415926
  Constant1 : Constant  Value=3.1415926
  Sum : Sum  Inputs=|++
  Switch : Switch
  Out1 : Outport
  wires:
  Switch/1 -> Sum/1
  Constant/1 -> Switch/1
  Sum/1 -> Out1/1
  In1/1 -> Sum/2, Switch/2
  Constant1/1 -> Switch/3

== system Pendulum/实验13  神经网络控制实验/  ==
  In1 : Inport
  Discrete Zero-Pole : DiscreteZeroPole  Poles=[0]  Gain=1  SampleTime=0.01
  Gain : Gain  Gain=1/0.01
  Out1 : Outport
  wires:
  Gain/1 -> Out1/1
  Discrete Zero-Pole/1 -> Gain/1
  In1/1 -> Discrete Zero-Pole/1

== system Pendulum/实验13  神经网络控制实验/   ==
  In1 : Inport
  Discrete Zero-Pole : DiscreteZeroPole  Poles=[0]  Gain=1  SampleTime=0.01
  Gain : Gain  Gain=1/0.01
  Out1 : Outport
  wires:
  Gain/1 -> Out1/1
  Discrete Zero-Pole/1 -> Gain/1
  In1/1 -> Discrete Zero-Pole/1

== system Pendulum/实验13  神经网络控制实验/如果角度大于0.25弧 度，让电机减速停止 ==
  In1 : Inport
  Action Port : ActionPort  ActionType=else
  S-Function : S-Function  FunctionName=SetStop  EnableBusSupport=off
  wires:
  In1/1 -> S-Function/1

== system Pendulum/实验13  神经网络控制实验/电机加速 ==
  In1 : Inport
  Action Port : ActionPort  ActionType=then
  Display : Display
  S-Function : S-Function  FunctionName=SetMotorAcc  EnableBusSupport=off
  wires:
  In1/1 -> S-Function/1
  S-Function/1 -> Display/1

== system Pendulum/实验13  神经网络控制实验/神经网络控制器 ==
  note: 误差反向传播神经网络
  note: 径向基函数神经网络
  In1 : Inport
  BP Neural Network : Subsystem
  Linear Transformation Operations 线性转换运算（还原数据） : S-Function  FunctionName=LTO  EnableBusSupport=off
  Manual Switch : ManualSwitch  CurrentSetting=0
  RBF Neural Network : Subsystem
  Out1 : Outport
  wires:
  RBF Neural Network/1("y{1}") -> Manual Switch/2
  BP Neural Network/1("y{1}") -> Manual Switch/1
  In1/1 -> RBF Neural Network/1("p{1}"), BP Neural Network/1("p{1}")
  Manual Switch/1 -> Linear Transformation Operations 线性转换运算（还原数据）/1
  Linear Transformation Operations 线性转换运算（还原数据）/1 -> Out1/1

== system Pendulum/实验13  神经网络控制实验/竖直向上为零角度 ==
  In1 : Inport
  Constant : Constant  Value=-3.1415926
  Constant1 : Constant  Value=3.1415926
  Sum : Sum  Inputs=|++
  Switch : Switch
  Out1 : Outport
  wires:
  Switch/1 -> Sum/1
  Constant/1 -> Switch/1
  Sum/1 -> Out1/1
  In1/1 -> Sum/2, Switch/2
  Constant1/1 -> Switch/3

== system Pendulum/实验2  根轨迹校正实验/如果角度大于0.25弧 度，让电机减速停止 ==
  In1 : Inport
  Action Port : ActionPort  ActionType=else
  S-Function : S-Function  FunctionName=SetStop  EnableBusSupport=off
  wires:
  In1/1 -> S-Function/1

== system Pendulum/实验2  根轨迹校正实验/电机加速 ==
  In1 : Inport
  Action Port : ActionPort  ActionType=then
  Display : Display
  S-Function : S-Function  FunctionName=SetMotorAcc  EnableBusSupport=off
  wires:
  In1/1 -> S-Function/1
  S-Function/1 -> Display/1

== system Pendulum/实验2  根轨迹校正实验/竖直向上为零角度 ==
  In1 : Inport
  Constant : Constant  Value=-3.1415926
  Constant1 : Constant  Value=3.1415926
  Sum : Sum  Inputs=|++
  Switch : Switch
  Out1 : Outport
  wires:
  Switch/1 -> Sum/1
  Constant/1 -> Switch/1
  Sum/1 -> Out1/1
  In1/1 -> Sum/2, Switch/2
  Constant1/1 -> Switch/3

== system Pendulum/实验3  频率响应校正实验/如果角度大于0.25弧 度，让电机减速停止 ==
  In1 : Inport
  Action Port : ActionPort  ActionType=else
  S-Function : S-Function  FunctionName=SetStop  EnableBusSupport=off
  wires:
  In1/1 -> S-Function/1

== system Pendulum/实验3  频率响应校正实验/电机加速 ==
  In1 : Inport
  Action Port : ActionPort  ActionType=then
  Display : Display
  S-Function : S-Function  FunctionName=SetMotorAcc  EnableBusSupport=off
  wires:
  In1/1 -> S-Function/1
  S-Function/1 -> Display/1

== system Pendulum/实验3  频率响应校正实验/竖直向上为零角度 ==
  In1 : Inport
  Constant : Constant  Value=-3.1415926
  Constant1 : Constant  Value=3.1415926
  Sum : Sum  Inputs=|++
  Switch : Switch
  Out1 : Outport
  wires:
  Switch/1 -> Sum/1
  Constant/1 -> Switch/1
  Sum/1 -> Out1/1
  In1/1 -> Sum/2, Switch/2
  Constant1/1 -> Switch/3

== system Pendulum/实验4  PID控制实验/只对摆杆角度施加控制 ==
  In1 : Inport
  PID1 : Subsystem  mask{Kp=30, Ki=0, Kd=2.5}
      mask help: PID校正器
      mask Display: disp('摆杆角度PID校正器')
  Out1 : Outport
  wires:
  In1/1 -> PID1/1(In1)
  PID1/1(Out1) -> Out1/1

== system Pendulum/实验4  PID控制实验/如果角度大于0.25弧 度，让电机减速停止 ==
  In1 : Inport
  Action Port : ActionPort  ActionType=else
  S-Function : S-Function  FunctionName=SetStop  EnableBusSupport=off
  wires:
  In1/1 -> S-Function/1

== system Pendulum/实验4  PID控制实验/对摆杆角度和小车 位置同时施加控制 ==
  In3 : Inport
  In2 : Inport  Port=2
  PID2 : Subsystem  mask{Kp=1.9, Ki=0.02, Kd=1.45}
      mask help: PID校正器
      mask Display: disp('小车位置PID校正器')
  PID3 : Subsystem  mask{Kp=4, Ki=0, Kd=0.5}
      mask help: PID校正器
      mask Display: disp('摆杆角度PID校正器')
  Out3 : Outport
  Out2 : Outport  Port=2
  wires:
  In2/1 -> PID3/1(In1)
  In3/1 -> PID2/1(In1)
  PID3/1(Out1) -> Out2/1
  PID2/1(Out1) -> Out3/1

== system Pendulum/实验4  PID控制实验/电机加速 ==
  In1 : Inport
  Action Port : ActionPort  ActionType=then
  Display : Display
  S-Function : S-Function  FunctionName=SetMotorAcc  EnableBusSupport=off
  wires:
  In1/1 -> S-Function/1
  S-Function/1 -> Display/1

== system Pendulum/实验4  PID控制实验/竖直向上为零角度 ==
  In1 : Inport
  Constant : Constant  Value=-3.1415926
  Constant1 : Constant  Value=3.1415926
  Sum : Sum  Inputs=|++
  Switch : Switch
  Out1 : Outport
  wires:
  Switch/1 -> Sum/1
  Constant/1 -> Switch/1
  Sum/1 -> Out1/1
  In1/1 -> Sum/2, Switch/2
  Constant1/1 -> Switch/3

== system Pendulum/实验5  状态空间极点配置控制实验/  ==
  In1 : Inport
  Discrete Zero-Pole : DiscreteZeroPole  Poles=[0]  Gain=1  SampleTime=0.01
  Gain : Gain  Gain=1/0.01
  Out1 : Outport
  wires:
  Gain/1 -> Out1/1
  Discrete Zero-Pole/1 -> Gain/1
  In1/1 -> Discrete Zero-Pole/1

== system Pendulum/实验5  状态空间极点配置控制实验/   ==
  In1 : Inport
  Discrete Zero-Pole : DiscreteZeroPole  Poles=[0]  Gain=1  SampleTime=0.01
  Gain : Gain  Gain=1/0.01
  Out1 : Outport
  wires:
  Gain/1 -> Out1/1
  Discrete Zero-Pole/1 -> Gain/1
  In1/1 -> Discrete Zero-Pole/1

== system Pendulum/实验5  状态空间极点配置控制实验/    ==
  In1 : Inport
  Gain : Gain  Gain=[K1 K2 K3 K4]  Multiplication=Matrix(K*u)
  Out1 : Outport
  wires:
  In1/1 -> Gain/1
  Gain/1 -> Out1/1

== system Pendulum/实验5  状态空间极点配置控制实验/如果角度大于0.25弧 度，让电机减速停止 ==
  In1 : Inport
  Action Port : ActionPort  ActionType=else
  S-Function : S-Function  FunctionName=SetStop  EnableBusSupport=off
  wires:
  In1/1 -> S-Function/1

== system Pendulum/实验5  状态空间极点配置控制实验/电机加速 ==
  In1 : Inport
  Action Port : ActionPort  ActionType=then
  Display : Display
  S-Function : S-Function  FunctionName=SetMotorAcc  EnableBusSupport=off
  wires:
  In1/1 -> S-Function/1
  S-Function/1 -> Display/1

== system Pendulum/实验5  状态空间极点配置控制实验/竖直向上为零角度 ==
  In1 : Inport
  Constant : Constant  Value=-3.1415926
  Constant1 : Constant  Value=3.1415926
  Sum : Sum  Inputs=|++
  Switch : Switch
  Out1 : Outport
  wires:
  Switch/1 -> Sum/1
  Constant/1 -> Switch/1
  Sum/1 -> Out1/1
  In1/1 -> Sum/2, Switch/2
  Constant1/1 -> Switch/3

== system Pendulum/实验6  线性二次最优(LQR)控制实验/  ==
  In1 : Inport
  Discrete Zero-Pole : DiscreteZeroPole  Poles=[0]  Gain=1  SampleTime=0.01
  Gain : Gain  Gain=1/0.01
  Out1 : Outport
  wires:
  Gain/1 -> Out1/1
  Discrete Zero-Pole/1 -> Gain/1
  In1/1 -> Discrete Zero-Pole/1

== system Pendulum/实验6  线性二次最优(LQR)控制实验/   ==
  In1 : Inport
  Discrete Zero-Pole : DiscreteZeroPole  Poles=[0]  Gain=1  SampleTime=0.01
  Gain : Gain  Gain=1/0.01
  Out1 : Outport
  wires:
  Gain/1 -> Out1/1
  Discrete Zero-Pole/1 -> Gain/1
  In1/1 -> Discrete Zero-Pole/1

== system Pendulum/实验6  线性二次最优(LQR)控制实验/如果角度大于0.25弧 度，让电机减速停止 ==
  In1 : Inport
  Action Port : ActionPort  ActionType=else
  S-Function : S-Function  FunctionName=SetStop  EnableBusSupport=off
  wires:
  In1/1 -> S-Function/1

== system Pendulum/实验6  线性二次最优(LQR)控制实验/电机加速 ==
  In1 : Inport
  Action Port : ActionPort  ActionType=then
  Display : Display
  S-Function : S-Function  FunctionName=SetMotorAcc  EnableBusSupport=off
  wires:
  In1/1 -> S-Function/1
  S-Function/1 -> Display/1

== system Pendulum/实验6  线性二次最优(LQR)控制实验/竖直向上为零角度 ==
  In1 : Inport
  Constant : Constant  Value=-3.1415926
  Constant1 : Constant  Value=3.1415926
  Sum : Sum  Inputs=|++
  Switch : Switch
  Out1 : Outport
  wires:
  Switch/1 -> Sum/1
  Constant/1 -> Switch/1
  Sum/1 -> Out1/1
  In1/1 -> Sum/2, Switch/2
  Constant1/1 -> Switch/3

== system Pendulum/实验6  线性二次最优(LQR)控制实验/线性二次最优控制器 ==
  In1 : Inport
  Gain : Gain  Gain=[K1 K2 K3 K4]  Multiplication=Matrix(K*u)
  Out1 : Outport
  wires:
  In1/1 -> Gain/1
  Gain/1 -> Out1/1

== system Pendulum/实验7  LQR控制（Bang_Bang自摆起）实验/  ==
  In1 : Inport
  Discrete Zero-Pole : DiscreteZeroPole  Poles=[0]  Gain=1  SampleTime=0.01
  Gain : Gain  Gain=1/0.01
  Out1 : Outport
  wires:
  Gain/1 -> Out1/1
  Discrete Zero-Pole/1 -> Gain/1
  In1/1 -> Discrete Zero-Pole/1

== system Pendulum/实验7  LQR控制（Bang_Bang自摆起）实验/   ==
  In1 : Inport
  Discrete Zero-Pole : DiscreteZeroPole  Poles=[0]  Gain=1  SampleTime=0.01
  Gain : Gain  Gain=1/0.01
  Out1 : Outport
  wires:
  Gain/1 -> Out1/1
  Discrete Zero-Pole/1 -> Gain/1
  In1/1 -> Discrete Zero-Pole/1

== system Pendulum/实验7  LQR控制（Bang_Bang自摆起）实验/        ==
  In1 : Inport
  Discrete Zero-Pole : DiscreteZeroPole  Poles=[0]  Gain=1  SampleTime=0.01
  Gain : Gain  Gain=1/0.01
  Out1 : Outport
  wires:
  Gain/1 -> Out1/1
  Discrete Zero-Pole/1 -> Gain/1
  In1/1 -> Discrete Zero-Pole/1

== system Pendulum/实验7  LQR控制（Bang_Bang自摆起）实验/电机加速 ==
  In1 : Inport
  Action Port : ActionPort  ActionType=then
  Display : Display
  S-Function : S-Function  FunctionName=SetMotorAcc  EnableBusSupport=off
  wires:
  In1/1 -> S-Function/1
  S-Function/1 -> Display/1

== system Pendulum/实验7  LQR控制（Bang_Bang自摆起）实验/竖直向上为零角度 ==
  In1 : Inport
  Constant : Constant  Value=-3.1415926
  Constant1 : Constant  Value=3.1415926
  Sum : Sum  Inputs=|++
  Switch : Switch
  Out1 : Outport
  wires:
  Switch/1 -> Sum/1
  Constant/1 -> Switch/1
  Sum/1 -> Out1/1
  In1/1 -> Sum/2, Switch/2
  Constant1/1 -> Switch/3

== system Pendulum/实验7  LQR控制（Bang_Bang自摆起）实验/线性二次最优控制器 ==
  In1 : Inport
  Gain : Gain  Gain=[K1 K2 K3 K4]  Multiplication=Matrix(K*u)
  Out1 : Outport
  wires:
  In1/1 -> Gain/1
  Gain/1 -> Out1/1

== system Pendulum/实验7  LQR控制（Bang_Bang自摆起）实验/自摆 ==
  " " : Inport
  "  " : Inport  Port=2
  "   " : Inport  Port=3
  Action Port : ActionPort  ActionType=else
  S-Function : S-Function  FunctionName=BangBangSwingUp  EnableBusSupport=off
      mask Display:
      | port_label('input',1,'ANG')
      | port_label('input',2,'VEL')
      | port_label('input',3,'ACC')
  wires:
  " "/1 -> S-Function/1
  "  "/1 -> S-Function/2
  "   "/1 -> S-Function/3

== system Pendulum/实验8  LQR控制（能量自摆起）实验/  ==
  In1 : Inport
  Discrete Zero-Pole : DiscreteZeroPole  Poles=[0]  Gain=1  SampleTime=0.01
  Gain : Gain  Gain=1/0.01
  Out1 : Outport
  wires:
  Gain/1 -> Out1/1
  Discrete Zero-Pole/1 -> Gain/1
  In1/1 -> Discrete Zero-Pole/1

== system Pendulum/实验8  LQR控制（能量自摆起）实验/   ==
  In1 : Inport
  Discrete Zero-Pole : DiscreteZeroPole  Poles=[0]  Gain=1  SampleTime=0.01
  Gain : Gain  Gain=1/0.01
  Out1 : Outport
  wires:
  Gain/1 -> Out1/1
  Discrete Zero-Pole/1 -> Gain/1
  In1/1 -> Discrete Zero-Pole/1

== system Pendulum/实验8  LQR控制（能量自摆起）实验/        ==
  In1 : Inport
  Discrete Zero-Pole : DiscreteZeroPole  Poles=[0]  Gain=1  SampleTime=0.01
  Gain : Gain  Gain=1/0.01
  Out1 : Outport
  wires:
  Gain/1 -> Out1/1
  Discrete Zero-Pole/1 -> Gain/1
  In1/1 -> Discrete Zero-Pole/1

== system Pendulum/实验8  LQR控制（能量自摆起）实验/电机加速 ==
  In1 : Inport
  Action Port : ActionPort  ActionType=then
  Display : Display
  S-Function : S-Function  FunctionName=SetMotorAcc  EnableBusSupport=off
  wires:
  In1/1 -> S-Function/1
  S-Function/1 -> Display/1

== system Pendulum/实验8  LQR控制（能量自摆起）实验/竖直向上为零角度 ==
  In1 : Inport
  Constant : Constant  Value=-3.1415926
  Constant1 : Constant  Value=3.1415926
  Sum : Sum  Inputs=|++
  Switch : Switch
  Out1 : Outport
  wires:
  Switch/1 -> Sum/1
  Constant/1 -> Switch/1
  Sum/1 -> Out1/1
  In1/1 -> Sum/2, Switch/2
  Constant1/1 -> Switch/3

== system Pendulum/实验8  LQR控制（能量自摆起）实验/线性二次最优控制器 ==
  In1 : Inport
  Gain : Gain  Gain=[K1 K2 K3 K4]  Multiplication=Matrix(K*u)
  Out1 : Outport
  wires:
  In1/1 -> Gain/1
  Gain/1 -> Out1/1

== system Pendulum/实验8  LQR控制（能量自摆起）实验/自摆 ==
  " " : Inport
  "  " : Inport  Port=2
  "   " : Inport  Port=3
  "      " : Inport  Port=4
  Action Port : ActionPort  ActionType=else
  能量自摆 : S-Function  FunctionName=EnergySwingUp  EnableBusSupport=off  mask(EnergySwingUp){}
      mask help:
      | 元创兴便携式倒立摆simulink模块：
      |
      | 能量自摆起算法
      | 输入参数有四个：
      | 1.摆杆角度
      | 2.摆杆速度
      | 3.调整系数
      | 4.输入速度
      mask Display:
      | disp('EnergySwingUp')
      | port_label('input',1,'ANG')
      | port_label('input',2,'VEL')
      | port_label('input',3,'RAT')
      | port_label('input',4,'ACC')
  wires:
  " "/1 -> 能量自摆/1
  "  "/1 -> 能量自摆/2
  "   "/1 -> 能量自摆/3
  "      "/1 -> 能量自摆/4

== system Pendulum/实验9  模糊控制实验/  ==
  In1 : Inport
  Discrete Zero-Pole : DiscreteZeroPole  Poles=[0]  Gain=1  SampleTime=0.01
  Gain : Gain  Gain=1/0.01
  Out1 : Outport
  wires:
  Gain/1 -> Out1/1
  Discrete Zero-Pole/1 -> Gain/1
  In1/1 -> Discrete Zero-Pole/1

== system Pendulum/实验9  模糊控制实验/   ==
  In1 : Inport
  Discrete Zero-Pole : DiscreteZeroPole  Poles=[0]  Gain=1  SampleTime=0.01
  Gain : Gain  Gain=1/0.01
  Out1 : Outport
  wires:
  Gain/1 -> Out1/1
  Discrete Zero-Pole/1 -> Gain/1
  In1/1 -> Discrete Zero-Pole/1

== system Pendulum/实验9  模糊控制实验/模糊逻辑控制 ==
  In1 : Inport
  Demux : Demux
  Fuzzy Logic Controller : fuzblock/Fuzzy Logic  Controller  fis=fuzzycontroller1
  Gain : Gain  Gain=[-10.000 37.2688]  Multiplication=Matrix(K*u) (u vector)
  Gain1 : Gain  Gain=39.5790
  Gain2 : Gain  Gain=[-7.4869 4.6349]  Multiplication=Matrix(K*u) (u vector)
  Gain3 : Gain  Gain=1/39.5790
  Mux : Mux  Inputs=2
  Mux1 : Mux  Inputs=2
  Mux2 : Mux  Inputs=2
  Out1 : Outport
  wires:
  Mux1/1 -> Gain2/1
  Gain/1 -> Mux2/1
  Gain2/1 -> Mux2/2
  Demux/3 -> Mux/2
  Gain1/1 -> Out1/1
  Gain3/1 -> Fuzzy Logic Controller/1
  Fuzzy Logic Controller/1 -> Gain1/1
  In1/1 -> Demux/1
  Mux2/1 -> Gain3/1
  Demux/1 -> Mux/1
  Demux/4 -> Mux1/2
  Demux/2 -> Mux1/1
  Mux/1 -> Gain/1

== system Pendulum/实验9  模糊控制实验/电机停止 ==
  In1 : Inport
  Action Port : ActionPort  ActionType=else
  S-Function : S-Function  FunctionName=SetStop  EnableBusSupport=off
  wires:
  In1/1 -> S-Function/1

== system Pendulum/实验9  模糊控制实验/电机加速 ==
  In1 : Inport
  Action Port : ActionPort  ActionType=then
  Display : Display
  S-Function : S-Function  FunctionName=SetMotorAcc  EnableBusSupport=off
  wires:
  In1/1 -> S-Function/1
  S-Function/1 -> Display/1

== system Pendulum/实验9  模糊控制实验/竖直向上为零角度 ==
  In1 : Inport
  Constant : Constant  Value=-3.1415926
  Constant1 : Constant  Value=3.1415926
  Sum : Sum  Inputs=|++
  Switch : Switch
  Out1 : Outport
  wires:
  Switch/1 -> Sum/1
  Constant/1 -> Switch/1
  Sum/1 -> Out1/1
  In1/1 -> Sum/2, Switch/2
  Constant1/1 -> Switch/3

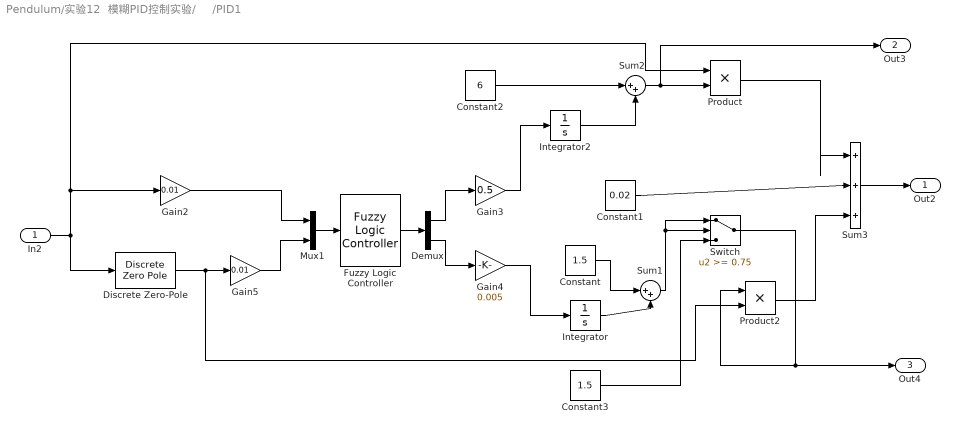
== system Pendulum/实验12  模糊PID控制实验/     /PID1 ==
  In2 : Inport
  Constant : Constant  Value=1.5
  Constant1 : Constant  Value=0.02
  Constant2 : Constant  Value=6
  Constant3 : Constant  Value=1.5
  Demux : Demux  Outputs=2
  Discrete Zero-Pole : DiscreteZeroPole  Poles=[0]  Gain=35  SampleTime=0.01
  Fuzzy Logic Controller : fuzblock/Fuzzy Logic  Controller  fis=fuzzypid
  Gain2 : Gain  Gain=0.01  SaturateOnIntegerOverflow=on  OutDataTypeStr=Inherit: Same as input  ParamDataTypeStr=Inherit: Same as input
  Gain3 : Gain  Gain=0.5  SaturateOnIntegerOverflow=on  OutDataTypeStr=Inherit: Same as input  ParamDataTypeStr=Inherit: Same as input
  Gain4 : Gain  Gain=0.005  SaturateOnIntegerOverflow=on  OutDataTypeStr=Inherit: Same as input  ParamDataTypeStr=Inherit: Same as input
  Gain5 : Gain  Gain=0.01  SaturateOnIntegerOverflow=on  OutDataTypeStr=Inherit: Same as input  ParamDataTypeStr=Inherit: Same as input
  Integrator : Integrator
  Integrator2 : Integrator
  Mux1 : Mux  Inputs=2
  Product : Product  SaturateOnIntegerOverflow=on  OutDataTypeStr=Inherit: Same as first input
  Product2 : Product  SaturateOnIntegerOverflow=on  OutDataTypeStr=Inherit: Same as first input
  Sum1 : Sum  Inputs=|++  SaturateOnIntegerOverflow=on
  Sum2 : Sum  Inputs=|++  SaturateOnIntegerOverflow=on
  Sum3 : Sum  Inputs=|+++  SaturateOnIntegerOverflow=on
  Switch : Switch  Threshold=0.75  SaturateOnIntegerOverflow=on
  Out2 : Outport
  Out3 : Outport  Port=2
  Out4 : Outport  Port=3
  wires:
  Sum3/1 -> Out2/1
  Discrete Zero-Pole/1 -> Gain5/1, Product2/2
  Switch/1 -> Out4/1, Product2/1
  Product2/1 -> Sum3/3
  In2/1 -> Discrete Zero-Pole/1, Gain2/1, Product/1
  Constant3/1 -> Switch/3
  Fuzzy Logic Controller/1 -> Demux/1
  Sum2/1 -> Out3/1, Product/2
  Gain5/1 -> Mux1/2
  Constant2/1 -> Sum2/1
  Constant/1 -> Sum1/1
  Mux1/1 -> Fuzzy Logic Controller/1
  Constant1/1 -> Sum3/2
  Integrator/1 -> Sum1/2
  Demux/1 -> Gain3/1
  Demux/2 -> Gain4/1
  Product/1 -> Sum3/1
  Sum1/1 -> Switch/2, Switch/1
  Gain3/1 -> Integrator2/1
  Gain2/1 -> Mux1/1
  Integrator2/1 -> Sum2/2
  Gain4/1 -> Integrator/1
